simulink model "sampleModel2010"  (R2023a)
settings: Solver=VariableStepAuto  StartTime=0.0  StopTime=10.0  RelTol=1e-3
libraries: hdlsllib x7, simulink x6
settings Model: Creator=user1  LastModifiedBy=user1

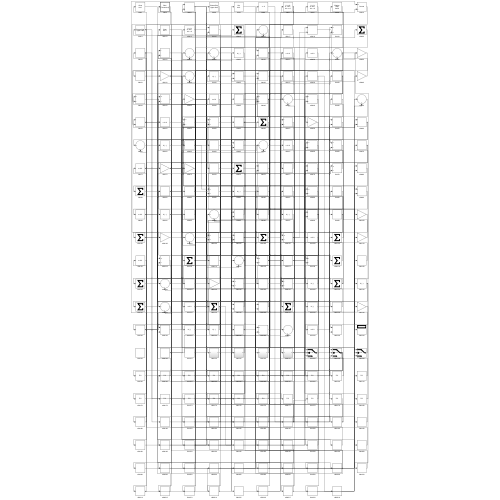
[thumbnail: Simulink's stored preview of the top-level diagram]
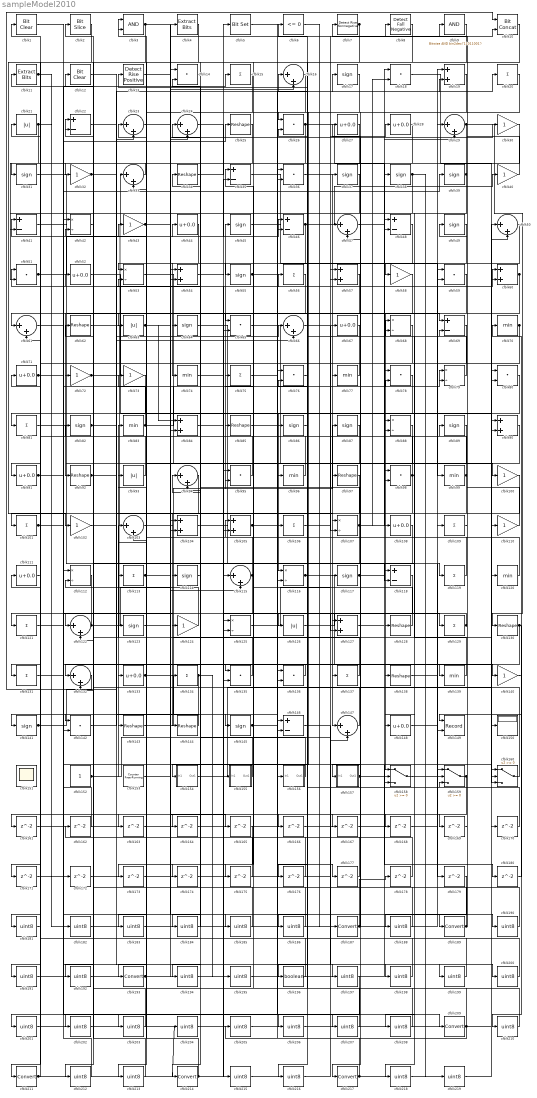
== system sampleModel2010 ==
  cfblk1 : simulink/Logic and Bit Operations/Bit Clear  iBit=0
      settings: LibrarySourceBlock=|
      | hdlsllib/Logic and Bit
      | Operations/Bit Clear
  cfblk10 : hdlsllib/Logic and Bit Operations/Bit Concat  numInputs=2
  cfblk{30,32,40,43,58,72..73,100,102,110,124,140} (12 alike) : Gain
  cfblk{15,20,56,75,81,101,106,109,113,119,121,129,131,134,137} (15 alike) : Sum  Inputs=+
  cfblk{16,23..24,29,33,47,50,61,66,94,103,115,122,132,147} (15 alike) : Sum  Inputs=|++
  cfblk{19,54,57,60,84,90,104..105,127} (9 alike) : Sum
  cfblk{42,53,68,79,88,107,112,116,125} (9 alike) : Product  Inputs=*/  RndMeth=Zero  SaturateOnIntegerOverflow=on
  cfblk{27..28,44,52,67,71,91,108,111,133,148} (11 alike) : Bias  Bias=0.0  SaturateOnIntegerOverflow=off
  cfblk11 : simulink/Logic and Bit Operations/Extract Bits  bitsToExtract=Upper half  numBits=8  bitIdxRange=[0 7]  outScalingMode=Preserve fixed-point scaling
      settings: LibrarySourceBlock=|
      | hdlsllib/Logic and Bit
      | Operations/Extract Bits
  cfblk{17,31,37..39,45,49,55,64,82,86..87,89,114,117,123,141,145} (18 alike) : Signum
  cfblk{22,35,41,46,48,69,118,146} (8 alike) : Sum  Inputs=+-
  cfblk12 : simulink/Logic and Bit Operations/Bit Clear  iBit=0
      settings: LibrarySourceBlock=|
      | hdlsllib/Logic and Bit
      | Operations/Bit Clear
  cfblk{70,74,77,83,96,99,120,139} (8 alike) : MinMax
  cfblk{21,63,93,126} (4 alike) : Abs  SaturateOnIntegerOverflow=off
  cfblk{25,34,62,85,92,97,128,130,138,143..144} (11 alike) : Reshape
  cfblk13 : hdlsllib/Logic and Bit Operations/Detect Rise Positive  vinit=0  OutDataTypeStr=boolean
  cfblk{14,18,26,36,51,59,65,76,78,80,95,98,135..136,142} (15 alike) : DotProduct  OutDataTypeStr=Inherit: Inherit via internal rule
  cfblk149 : Record  FileSettingsInternal="{\"entries\":[{\"content\":{\"excelSettings\":{\"content\":{},\"type\":\"Streamout.ExcelSettings\"}},\"type\":\"Streamout.FileSettingStorage\",\"uuid\":\"\"}],\"packageUris\":[\"http:\\/\\/schema.mathworks.com\\/mf0\\/streamout_blocks\\/R2020a\"],\"version\":\"1.0\"}"  Layout=[1 1]  SignalsInternal="{\"entries\":[{\"content\":{\"signals\":[{\"content\":{\"blockPath\":[],\"dimensions\":[1],\"domain\":\"\",\"lineColor\":\"#a2142f\",\"plots\":[1],\"port\":1,\"signalID\":5917,\"signalName\":\"XY Graph:1\"},\"type\":\"RecordBlkView.Signal\",\"uuid\":\"\"},{\"content\":{\"blockPath\":[],\"dimensions\":[1],\"domain\":\"\",\"lineColor\":\"#139fff\",\"plots\":[1],\"port\":2,\"signalID\":5920,\"signalName\":\"XY Graph:2\"},\"type\":\"RecordBlkView.Signal\",\"uuid\":\"\"}]},\"type\":\"RecordBlkView.InputSignals\",\"uuid\":\"\"}],\"packageUris\":[\"http:\\/\\/schema.mathworks.com\\/mf0\\/streamout_blocks\\/R2020a\"],\"version\":\"1.0\"}"  VisualizationBindings="{\"xyplotplugin\":{\"info\":[{\"series\":[{\"bindingParametersList\":[{\"parameter\":\"X-Axis\",\"signalID\":5917,\"signalName\":\"XY Graph:1\"},{\"parameter\":\"Y-Axis\",\"signalID\":5920,\"signalName\":\"XY Graph:2\"}],\"seriesID\":54583}],\"subplotID\":1}]}}"  CompatibilityTag=XY  st=-1
  cfblk150 : Display
  cfblk151 : Scope
      settings: Floating=on
  cfblk152 : Constant  SampleTime=-1
  cfblk153 : hdlsllib/Sources/Counter Free-Running  NumBits=16  tsamp=-1
  cfblk154 : Subsystem
      settings: LibrarySourceBlock=|
      | hdlsllib/Ports &
      | Subsystems/Subsystem
  cfblk155 : Subsystem
      settings: LibrarySourceBlock=|
      | hdlsllib/Ports &
      | Subsystems/Subsystem
  cfblk156 : Subsystem
      settings: LibrarySourceBlock=|
      | hdlsllib/Ports &
      | Subsystems/Subsystem
  cfblk157 : Subsystem
      settings: LibrarySourceBlock=|
      | hdlsllib/Ports &
      | Subsystems/Subsystem
  cfblk158 : Switch  SaturateOnIntegerOverflow=off  InputSameDT=off
  cfblk159 : Switch  SaturateOnIntegerOverflow=off  InputSameDT=off
  cfblk160 : Switch  SaturateOnIntegerOverflow=off  InputSameDT=off
  cfblk{161..180} (20 alike) : Delay  SampleTime=1
  cfblk{181..186,188,190..192,194..195,197..208,210,212..213,215..216,218..219} (31 alike) : DataTypeConversion  OutDataTypeStr=uint8  SaturateOnIntegerOverflow=off  RndMeth=Floor
  cfblk{187,189,193,209,211,214,217} (7 alike) : DataTypeConversion  SaturateOnIntegerOverflow=off  RndMeth=Floor
  cfblk196 : DataTypeConversion  OutDataTypeStr=boolean  SaturateOnIntegerOverflow=off  RndMeth=Floor
  cfblk2 : hdlsllib/Logic and Bit Operations/Bit Slice  lidx=7  ridx=0
  cfblk3 : Logic  AllPortsSameDT=off  OutDataTypeStr=boolean
  cfblk4 : simulink/Logic and Bit Operations/Extract Bits  bitsToExtract=Upper half  numBits=8  bitIdxRange=[0 7]  outScalingMode=Preserve fixed-point scaling
      settings: LibrarySourceBlock=|
      | hdlsllib/Logic and Bit
      | Operations/Extract Bits
  cfblk5 : simulink/Logic and Bit Operations/Bit Set  iBit=0
      settings: LibrarySourceBlock=|
      | hdlsllib/Logic and Bit
      | Operations/Bit Set
  cfblk6 : hdlsllib/Logic and Bit Operations/Compare To Zero  relop=<=  OutDataTypeStr=boolean
  cfblk7 : hdlsllib/Logic and Bit Operations/Detect Rise Nonnegative  vinit=0  OutDataTypeStr=boolean
  cfblk8 : hdlsllib/Logic and Bit Operations/Detect Fall Negative  vinit=0  OutDataTypeStr=boolean
  cfblk9 : simulink/Logic and Bit Operations/Bitwise Operator  logicop=AND  UseBitMask=on  BitMask=bin2dec('11011001')  BitMaskRealWorld=Stored Integer
      settings: LibrarySourceBlock=|
      | hdlsllib/Logic and Bit
      | Operations/Bitwise
      | Operator
  wires:
  cfblk56/1 -> cfblk61/1
  cfblk60/1 -> cfblk158/1, cfblk196/1
  cfblk9/1 -> cfblk132/1
  cfblk20/1 -> cfblk154/1(In1)
  cfblk31/1 -> cfblk119/1
  cfblk2/1 -> cfblk102/1
  cfblk58/1 -> cfblk92/1
  cfblk152/1 -> cfblk33/1, cfblk8/1
  cfblk119/1 -> cfblk33/2
  cfblk10/1 -> cfblk61/2
  cfblk144/1 -> cfblk141/1
  cfblk137/1 -> cfblk83/1
  cfblk91/1 -> cfblk123/1, cfblk185/1
  cfblk57/1 -> cfblk214/1
  cfblk156/1(Out1) -> cfblk24/1
  cfblk45/1 -> cfblk58/1
  cfblk103/1 -> cfblk45/1
  cfblk36/1 -> cfblk147/1
  cfblk112/1 -> cfblk211/1
  cfblk131/1 -> cfblk39/1
  cfblk148/1 -> cfblk109/1
  cfblk116/1 -> cfblk140/1, cfblk28/1
  cfblk132/1 -> cfblk10/1
  cfblk37/1 -> cfblk55/1
  cfblk95/1 -> cfblk3/1
  cfblk105/1 -> cfblk136/2, cfblk158/2
  cfblk23/1 -> cfblk117/1
  cfblk124/1 -> cfblk62/1
  cfblk29/1 -> cfblk130/1, cfblk126/1, cfblk103/2
  cfblk79/1 -> cfblk13/1
  cfblk134/1 -> cfblk142/2, cfblk195/1
  cfblk88/1 -> cfblk113/1
  cfblk130/1 -> cfblk149/1, cfblk163/1
  cfblk143/1 -> cfblk87/1
  cfblk70/1 -> cfblk77/1, cfblk157/1(In1)
  cfblk11/1 -> cfblk81/1, cfblk172/1
  cfblk98/1 -> cfblk144/1, cfblk148/1, cfblk82/1
  cfblk46/1 -> cfblk40/1, cfblk135/2, cfblk213/1
  cfblk67/1 -> cfblk131/1
  cfblk52/1 -> cfblk116/1
  cfblk96/1 -> cfblk23/1
  cfblk157/1(Out1) -> cfblk60/1, cfblk180/1
  cfblk89/1 -> cfblk96/1
  cfblk33/1 -> cfblk32/1
  cfblk77/1 -> cfblk72/1
  cfblk30/1 -> cfblk53/1
  cfblk7/1 -> cfblk135/1, cfblk26/1
  cfblk92/1 -> cfblk107/1, cfblk66/2
  cfblk64/1 -> cfblk159/2
  cfblk16/1 -> cfblk143/1
  cfblk82/1 -> cfblk60/2, cfblk19/2
  cfblk66/1 -> cfblk107/2
  cfblk139/1 -> cfblk68/1
  cfblk126/1 -> cfblk128/1
  cfblk39/1 -> cfblk31/1, cfblk41/2, cfblk166/1, cfblk208/1
  cfblk53/1 -> cfblk150/1
  cfblk153/1 -> cfblk189/1
  cfblk44/1 -> cfblk74/1
  cfblk155/1(Out1) -> cfblk34/1
  cfblk106/1 -> cfblk67/1
  cfblk72/1 -> cfblk38/1, cfblk160/1, cfblk105/2
  cfblk125/1 -> cfblk37/1
  cfblk117/1 -> cfblk68/2, cfblk29/2
  cfblk142/1 -> cfblk44/1
  cfblk113/1 -> cfblk4/1, cfblk46/1
  cfblk129/1 -> cfblk122/1, cfblk9/1
  cfblk135/1 -> cfblk11/1
  cfblk154/1(Out1) -> cfblk120/1
  cfblk141/1 -> cfblk23/2, cfblk78/2, cfblk207/1
  cfblk65/1 -> cfblk100/1
  cfblk17/1 -> cfblk114/1
  cfblk145/1 -> cfblk86/1, cfblk105/1
  cfblk120/1 -> cfblk41/1
  cfblk18/1 -> cfblk90/1
  cfblk13/1 -> cfblk10/2
  cfblk21/1 -> cfblk51/2, cfblk182/1
  cfblk61/1 -> cfblk15/1
  cfblk121/1 -> cfblk25/1
  cfblk24/1 -> cfblk129/1
  cfblk32/1 -> cfblk139/1, cfblk158/3
  cfblk90/1 -> cfblk127/1
  cfblk158/1 -> cfblk19/1
  cfblk47/1 -> cfblk98/2
  cfblk128/1 -> cfblk75/1
  cfblk3/1 -> cfblk104/1, cfblk132/2, cfblk165/1
  cfblk41/1 -> cfblk64/1
  cfblk104/1 -> cfblk149/2
  cfblk107/1 -> cfblk18/2, cfblk51/1, cfblk79/2, cfblk176/1
  cfblk73/1 -> cfblk91/1
  cfblk159/1 -> cfblk169/1, cfblk191/1, cfblk202/1
  cfblk99/1 -> cfblk53/2, cfblk118/1, cfblk216/1
  cfblk50/1 -> cfblk217/1
  cfblk43/1 -> cfblk30/1, cfblk118/2, cfblk88/2
  cfblk26/1 -> cfblk108/1, cfblk173/1
  cfblk102/1 -> cfblk66/1
  cfblk22/1 -> cfblk145/1
  cfblk87/1 -> cfblk116/2
  cfblk40/1 -> cfblk7/1
  cfblk101/1 -> cfblk124/1, cfblk160/3
  cfblk84/1 -> cfblk56/1
  cfblk115/1 -> cfblk42/2, cfblk142/1
  cfblk83/1 -> cfblk79/1, cfblk73/1
  cfblk63/1 -> cfblk16/2, cfblk84/1
  cfblk62/1 -> cfblk69/1
  cfblk49/1 -> cfblk138/1
  cfblk48/1 -> cfblk193/1
  cfblk94/1 -> cfblk104/2
  cfblk85/1 -> cfblk209/1
  cfblk81/1 -> cfblk97/1
  cfblk42/1 -> cfblk22/1
  cfblk123/1 -> cfblk115/2
  cfblk93/1 -> cfblk21/1
  cfblk136/1 -> cfblk133/1
  cfblk71/1 -> cfblk137/1, cfblk160/2
  cfblk55/1 -> cfblk17/1, cfblk20/1, cfblk175/1
  cfblk110/1 -> cfblk49/1
  cfblk4/1 -> cfblk63/1
  cfblk27/1 -> cfblk65/1
  cfblk6/1 -> cfblk187/1
  cfblk15/1 -> cfblk94/2
  cfblk122/1 -> cfblk121/1, cfblk84/2
  cfblk147/1 -> cfblk35/1
  cfblk34/1 -> cfblk5/1
  cfblk35/1 -> cfblk99/1
  cfblk160/1 -> cfblk2/1
  cfblk75/1 -> cfblk36/2
  cfblk38/1 -> cfblk125/2, cfblk219/1
  cfblk133/1 -> cfblk156/1(In1), cfblk90/2
  cfblk118/1 -> cfblk127/2
  cfblk51/1 -> cfblk35/2, cfblk134/1
  cfblk28/1 -> cfblk106/1
  cfblk127/1 -> cfblk78/1
  cfblk25/1 -> cfblk101/1
  cfblk109/1 -> cfblk89/1
  cfblk111/1 -> cfblk161/1
  cfblk161/1 -> cfblk98/1
  cfblk162/1 -> cfblk42/1
  cfblk163/1 -> cfblk24/2
  cfblk78/1 -> cfblk164/1
  cfblk164/1 -> cfblk29/1
  cfblk166/1 -> cfblk47/1
  cfblk19/1 -> cfblk167/1
  cfblk167/1 -> cfblk88/1
  cfblk100/1 -> cfblk168/1
  cfblk168/1 -> cfblk159/1
  cfblk169/1 -> cfblk69/2
  cfblk170/1 -> cfblk16/1
  cfblk97/1 -> cfblk171/1
  cfblk171/1 -> cfblk147/2
  cfblk173/1 -> cfblk46/2
  cfblk114/1 -> cfblk174/1
  cfblk174/1 -> cfblk115/1
  cfblk175/1 -> cfblk122/2
  cfblk176/1 -> cfblk103/1
  cfblk5/1 -> cfblk177/1
  cfblk177/1 -> cfblk136/1
  cfblk178/1 -> cfblk22/2
  cfblk138/1 -> cfblk179/1
  cfblk180/1 -> cfblk70/1
  cfblk59/1 -> cfblk181/1
  cfblk181/1 -> cfblk71/1
  cfblk182/1 -> cfblk59/1
  cfblk165/1 -> cfblk183/1
  cfblk183/1 -> cfblk59/2
  cfblk14/1 -> cfblk184/1
  cfblk184/1 -> cfblk94/1
  cfblk185/1 -> cfblk14/1
  cfblk86/1 -> cfblk186/1
  cfblk186/1 -> cfblk14/2
  cfblk187/1 -> cfblk178/1, cfblk95/2, cfblk52/1, cfblk47/2
  cfblk69/1 -> cfblk188/1
  cfblk188/1 -> cfblk6/1
  cfblk189/1 -> cfblk26/2, cfblk159/3
  cfblk54/1 -> cfblk190/1
  cfblk190/1 -> cfblk27/1
  cfblk191/1 -> cfblk54/1
  cfblk108/1 -> cfblk192/1
  cfblk192/1 -> cfblk54/2
  cfblk193/1 -> cfblk65/2, cfblk155/1(In1)
  cfblk8/1 -> cfblk194/1
  cfblk194/1 -> cfblk48/1
  cfblk195/1 -> cfblk48/2
  cfblk196/1 -> cfblk12/1
  cfblk12/1 -> cfblk197/1
  cfblk1/1 -> cfblk198/1
  cfblk198/1 -> cfblk93/1
  cfblk172/1 -> cfblk199/1
  cfblk199/1 -> cfblk1/1
  cfblk146/1 -> cfblk200/1
  cfblk200/1 -> cfblk18/1
  cfblk197/1 -> cfblk201/1
  cfblk201/1 -> cfblk146/1
  cfblk202/1 -> cfblk146/2
  cfblk80/1 -> cfblk203/1
  cfblk203/1 -> cfblk162/1
  cfblk204/1 -> cfblk80/1
  cfblk205/1 -> cfblk80/2
  cfblk76/1 -> cfblk206/1
  cfblk206/1 -> cfblk170/1
  cfblk207/1 -> cfblk76/1
  cfblk208/1 -> cfblk76/2
  cfblk209/1 -> cfblk205/1, cfblk95/1, cfblk3/2
  cfblk140/1 -> cfblk210/1
  cfblk210/1 -> cfblk85/1
  cfblk211/1 -> cfblk204/1, cfblk111/1
  cfblk68/1 -> cfblk212/1
  cfblk212/1 -> cfblk112/1
  cfblk213/1 -> cfblk112/2
  cfblk214/1 -> cfblk125/1, cfblk43/1
  cfblk74/1 -> cfblk215/1
  cfblk215/1 -> cfblk57/1
  cfblk216/1 -> cfblk57/2
  cfblk217/1 -> cfblk110/1, cfblk36/1
  cfblk179/1 -> cfblk218/1
  cfblk218/1 -> cfblk50/1
  cfblk219/1 -> cfblk50/2

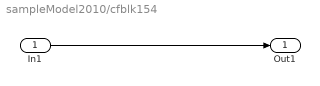
== system sampleModel2010/cfblk154 ==
  In1 : Inport
  Out1 : Outport
  wires:
  In1/1 -> Out1/1

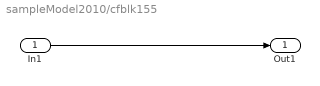
== system sampleModel2010/cfblk155 ==
  In1 : Inport
  Out1 : Outport
  wires:
  In1/1 -> Out1/1

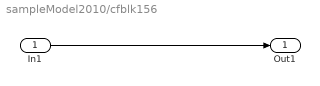
== system sampleModel2010/cfblk156 ==
  In1 : Inport
  Out1 : Outport
  wires:
  In1/1 -> Out1/1

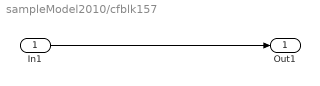
== system sampleModel2010/cfblk157 ==
  In1 : Inport
  Out1 : Outport
  wires:
  In1/1 -> Out1/1
